simulink model "full_state_linearized_model_with_observer"  (R2024b)
settings: Solver=VariableStepAuto  StartTime=0.0  StopTime=100  FixedStep=1e-3  RelTol=1e-4
undefined symbols (not defined in the file): A, B, C, K_L, K_lqr
settings Model: Creator=pedro  LastModifiedBy=pedro

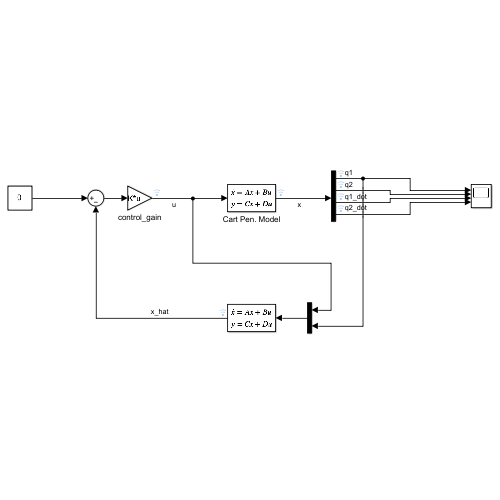
[thumbnail: Simulink's stored preview of the top-level diagram]
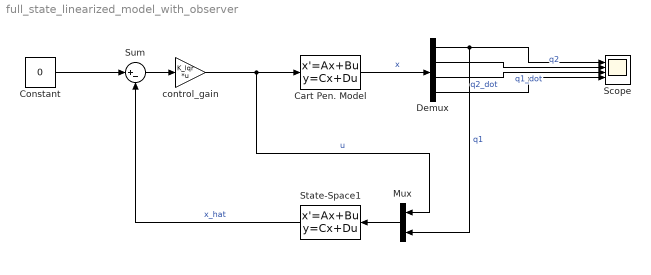
== system full_state_linearized_model_with_observer ==
  Cart Pen. Model : StateSpace  A=A  B=B  C=eye(4,4)  D=zeros(4,1)  InitialCondition=deg2rad(10)
  Constant : Constant  Value=0
  Demux : Demux
  Mux : Mux  Inputs=2
  Scope : Scope  NumInputPorts=4
  State-Space1 : StateSpace  A=A-K_L*C  B=[B K_L]  C=eye(4)  D=0*[B K_L]  InitialCondition=0
  Sum : Sum  Inputs=|+-
  control_gain : Gain  Gain=K_lqr  Multiplication=Matrix(K*u)
  wires:
  Cart Pen. Model/1 -> Demux/1  "x"
  Demux/1 -> Mux/2, Scope/1  "q1"
  Demux/2 -> Scope/2  "q2"
  Demux/3 -> Scope/3  "q1_dot"
  Demux/4 -> Scope/4  "q2_dot"
  Constant/1 -> Sum/1
  control_gain/1 -> Mux/1, Cart Pen. Model/1  "u"
  Sum/1 -> control_gain/1
  Mux/1 -> State-Space1/1
  State-Space1/1 -> Sum/2  "x_hat"
